simulink model "fish_deboning12"  (R2021a)
settings: Solver=VariableStepAuto  StartTime=0.0  StopTime=10.0  RelTol=1e-3  AbsTol=1e-3
libraries: fl_lib x47, ee_lib x44, nesl_utility x5
settings Model: Creator=Shivu  LastModifiedBy=Shivu
settings SolverCC: AutoScaleAbsTol=off  AlgebraicLoopSolver=TrustRegion
settings DebuggingCC: SymbolicDimsDataTypeCodeGenerationDiagnostic=none  SFMachineParentedDataDiag=warning
settings SFSimCC: CustomCodeUndefinedFunction=UseInterfaceOnly
settings SimscapeCC: SimscapeLogType=all  SimscapeLogSimulationStatistics=on  SimscapeLogDataHistory=10000

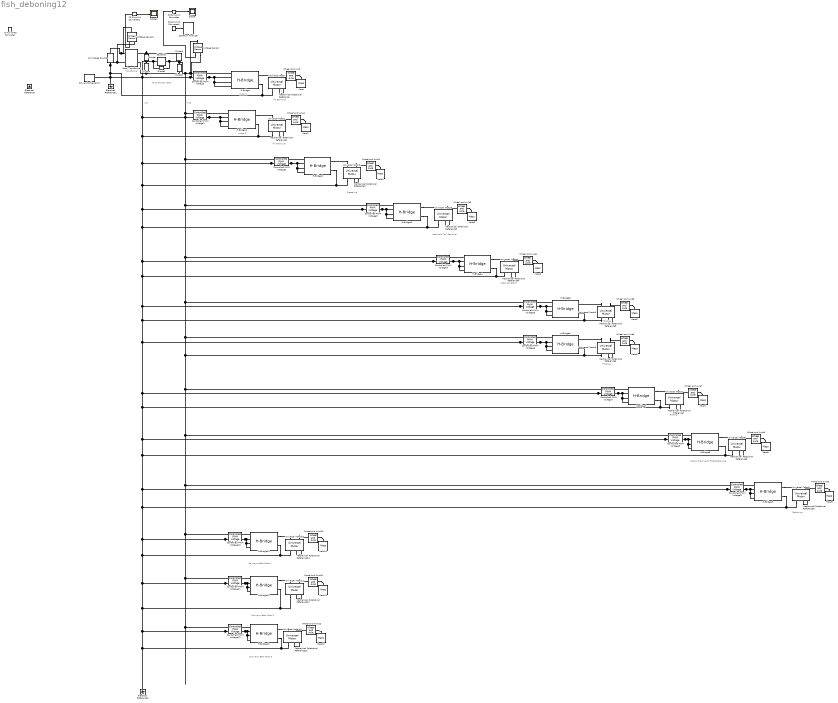
== system fish_deboning12 ==
  note: Conveyor Belt Motor 3
  note: Conveyor Belt Motor 2
  note: Conveyor Belt Motor 1
  note: Deboning
  note: Option flipping for Fillet/Deboning
  note: Gutting
  note: Filleting
  note: Filleting
  note: Head Collection
  note: Head and Tail Removal
  note: Descaling
  note: Fin Removal
  note: Fin Removal
  note: motor 2
  note: motor 1
  note: Transformer
  note: AC to DC Convertor
  note: +VE
  note: -VE
  AC Voltage Source : fl_lib/Electrical/Electrical Sources/AC Voltage Source  amp=230 V  shift=0 deg  frequency=50 Hz  omega=0 rad/s
  Capacitor : fl_lib/Electrical/Electrical Elements/Capacitor  c=4700 uF  r=1e-6 Ohm  g=0 1/Ohm  i_specify=off  i_priority=None  i=0 A  i_nominal_specify=off  i_nominal_unit=A  i_nominal_value=1  v_specify=on  v_priority=High  v=50 V  v_nominal_specify=off  v_nominal_unit=V  v_nominal_value=1  vc_specify=off  vc_priority=Low  vc=0 V  vc_nominal_specify=off  vc_nominal_unit=V  vc_nominal_value=1
  Controlled PWM Voltage{,1..12} (13 alike) : ee_lib/Integrated Circuits/Controlled PWM Voltage  F=1000 Hz  TD=0 s  pulse_width_offset=0 s  pulse_min=0 s  Vmin=0 V  Vmax=230 V  Vm=5 V  pwm_or_av=2  event_type=1  sample_time=1e-6 s  u_min=0  u_max=1
  Diode{,2..4} (4 alike) : ee_lib/Semiconductors & Converters/Diode  ModelType=ee.enum.diode.modelType.pwl  IfMat=[.07, .12, .19, 1.75, 4.24, 7.32, 11.2; .16, .3, .72, 2.14, 4.02, 6.35, 9.12] A  TjVec=[25, 125] degC  VfVec=[.5, .7, .9, 1.3, 1.7, 2.1, 2.5] V  Vf=1.1 V  Ron=0.3 Ohm  Goff=1e-8 S  prmExp=ee.enum.diode.expParam.useTwo  I12=[.0137, .545] A  V12=[.6, .7] V  IS=1e-12 A  ec=1  I1=0.0137 A  V1=0.6 V  RS=0 Ohm  Tmeas=25 degC  N_series=1  N_parallel=1  Rz=0.3 Ohm  BV=inf V  C_param=ee.enum.diode.capParam.fixed  CJ=5 pF  CJ0=5 pF  VJ=1 V  Mgrad=0.5  Vvec=[.1, 10, 100] V  Cvec=[3.5, 1, .4] pF  FC=0.5  Q_param=ee.enum.diode.recoveryParam.off  iRM=-7.15 A  iF=4 A  didt=-750 A/us  trr_factor=3  trr=115 ns  Qrr=150 s*nA  TT=50 ns  tau=100 ns  T_param=ee.enum.diode.temperatureParam.off  IS_T2=1.25e-7 A  I1_T2=0.245 A  V1_T2=0.5 V  Tmeas2=125 degC  EG_param=ee.enum.diode.egapParam.material_si  EG=1.11 eV  XTI_param=ee.enum.diode.xtiParam.pn  XTI=3  dBVdT=0 V/K  enable_faults=ee.enum.faults.faultEnable.no  fault_action=ee.enum.faults.faultAction.none  fault_types=ee.enum.diode.faults.open  tau_fault=1e-3 s  IfMat_faulted=[.07, .12, .19, 1.75, 4.24, 7.32, 11.2; .16, .3, .72, 2.14, 4.02, 6.35, 9.12] A  VfVec_faulted=[.5, .7, .9, 1.3, 1.7, 2.1, 2.5] V  Ropen_faulted=1000 Ohm  Gshort_faulted=1000 1/Ohm  Vf_faulted=0.6 V  Ron_faulted=0.3 Ohm  Goff_faulted=1e-8 S  I12_faulted=[.0137, .545] A  V12_faulted=[.6, .7] V  IS_faulted=1e-12 A  ec_faulted=1  I1_faulted=0.0137 A  V1_faulted=0.6 V  RS_faulted=0 Ohm  Rz_faulted=0.3 Ohm  BV_faulted=inf V  Cscale_faulted=100  enable_temporal_fault=ee.enum.faults.faultEnable.no  t_fault=inf s  enable_behavioral_fault=ee.enum.faults.faultEnable.no  max_permissible_voltage=inf V  n_fail_on_voltage=1  max_permissible_current=inf A  t_fail_on_current=1 s  max_permissible_dVdt=inf V/s  Tdevice=25 degC  i_specify=off  i_priority=None  i=0 A  i_nominal_specify=off  i_nominal_unit=A  i_nominal_value=1  v_specify=off  v_priority=None  v=0 V  v_nominal_specify=off  v_nominal_unit=V  v_nominal_value=1  i_diode_specify=off  i_diode_priority=None  i_diode=0 A  i_diode_nominal_specify=off  i_diode_nominal_unit=A  i_diode_nominal_value=1  v_diode_specify=off  v_diode_priority=None  v_diode=0 V  v_diode_nominal_specify=off  v_diode_nominal_unit=V  v_diode_nominal_value=1  i_capacitor_specify=off  i_capacitor_priority=None  i_capacitor=0 A  i_capacitor_nominal_specify=off  i_capacitor_nominal_unit=A  i_capacitor_nominal_value=1  v_capacitor_specify=off  v_capacitor_priority=None  v_capacitor=0 V  v_capacitor_nominal_specify=off  v_capacitor_nominal_unit=V  v_capacitor_nominal_value=1  power_dissipated_specify=off  power_dissipated_priority=None  power_dissipated=0 W  power_dissipated_nominal_specify=off  power_dissipated_nominal_unit=W  power_dissipated_nominal_value=1  max_permissible_temperature=inf K  t_fail_on_temperature=1 s  thermal_network_parameterization=ee.enum.thermalNetworkTopology.cauer  Rth=[0, 10] K/W  Rth_Foster=[4, 6] K/W  thermal_mass_parameterization=ee.enum.thermalNetwork.timeconstant  thermal_mass=[0, 1] J/K  thermal_mass_Foster=[1.5, 3] J/K  thermal_time_constant=[0, 10] s  thermal_time_constant_Foster=[6, 18] s  thermal_mass_initial_temperatures=[25, 25] degC
  Diode1 : ee_lib/Semiconductors & Converters/Diode  ModelType=ee.enum.diode.modelType.pwl  IfMat=[.07, .12, .19, 1.75, 4.24, 7.32, 11.2; .16, .3, .72, 2.14, 4.02, 6.35, 9.12] A  TjVec=[25, 125] degC  VfVec=[.5, .7, .9, 1.3, 1.7, 2.1, 2.5] V  Vf=0.6 V  Ron=0.3 Ohm  Goff=1e-8 S  prmExp=ee.enum.diode.expParam.useTwo  I12=[.0137, .545] A  V12=[.6, .7] V  IS=1e-12 A  ec=1  I1=0.0137 A  V1=0.6 V  RS=0 Ohm  Tmeas=25 degC  N_series=1  N_parallel=1  Rz=0.3 Ohm  BV=inf V  C_param=ee.enum.diode.capParam.fixed  CJ=5 pF  CJ0=5 pF  VJ=1 V  Mgrad=0.5  Vvec=[.1, 10, 100] V  Cvec=[3.5, 1, .4] pF  FC=0.5  Q_param=ee.enum.diode.recoveryParam.off  iRM=-7.15 A  iF=4 A  didt=-750 A/us  trr_factor=3  trr=115 ns  Qrr=150 s*nA  TT=50 ns  tau=100 ns  T_param=ee.enum.diode.temperatureParam.off  IS_T2=1.25e-7 A  I1_T2=0.245 A  V1_T2=0.5 V  Tmeas2=125 degC  EG_param=ee.enum.diode.egapParam.material_si  EG=1.11 eV  XTI_param=ee.enum.diode.xtiParam.pn  XTI=3  dBVdT=0 V/K  enable_faults=ee.enum.faults.faultEnable.no  fault_action=ee.enum.faults.faultAction.none  fault_types=ee.enum.diode.faults.open  tau_fault=1e-3 s  IfMat_faulted=[.07, .12, .19, 1.75, 4.24, 7.32, 11.2; .16, .3, .72, 2.14, 4.02, 6.35, 9.12] A  VfVec_faulted=[.5, .7, .9, 1.3, 1.7, 2.1, 2.5] V  Ropen_faulted=1000 Ohm  Gshort_faulted=1000 1/Ohm  Vf_faulted=0.6 V  Ron_faulted=0.3 Ohm  Goff_faulted=1e-8 S  I12_faulted=[.0137, .545] A  V12_faulted=[.6, .7] V  IS_faulted=1e-12 A  ec_faulted=1  I1_faulted=0.0137 A  V1_faulted=0.6 V  RS_faulted=0 Ohm  Rz_faulted=0.3 Ohm  BV_faulted=inf V  Cscale_faulted=100  enable_temporal_fault=ee.enum.faults.faultEnable.no  t_fault=inf s  enable_behavioral_fault=ee.enum.faults.faultEnable.no  max_permissible_voltage=inf V  n_fail_on_voltage=1  max_permissible_current=inf A  t_fail_on_current=1 s  max_permissible_dVdt=inf V/s  Tdevice=25 degC  i_specify=off  i_priority=None  i=0 A  i_nominal_specify=off  i_nominal_unit=A  i_nominal_value=1  v_specify=off  v_priority=None  v=0 V  v_nominal_specify=off  v_nominal_unit=V  v_nominal_value=1  i_diode_specify=off  i_diode_priority=None  i_diode=0 A  i_diode_nominal_specify=off  i_diode_nominal_unit=A  i_diode_nominal_value=1  v_diode_specify=off  v_diode_priority=None  v_diode=0 V  v_diode_nominal_specify=off  v_diode_nominal_unit=V  v_diode_nominal_value=1  i_capacitor_specify=off  i_capacitor_priority=None  i_capacitor=0 A  i_capacitor_nominal_specify=off  i_capacitor_nominal_unit=A  i_capacitor_nominal_value=1  v_capacitor_specify=off  v_capacitor_priority=None  v_capacitor=0 V  v_capacitor_nominal_specify=off  v_capacitor_nominal_unit=V  v_capacitor_nominal_value=1  power_dissipated_specify=off  power_dissipated_priority=None  power_dissipated=0 W  power_dissipated_nominal_specify=off  power_dissipated_nominal_unit=W  power_dissipated_nominal_value=1  max_permissible_temperature=inf K  t_fail_on_temperature=1 s  thermal_network_parameterization=ee.enum.thermalNetworkTopology.cauer  Rth=[0, 10] K/W  Rth_Foster=[4, 6] K/W  thermal_mass_parameterization=ee.enum.thermalNetwork.timeconstant  thermal_mass=[0, 1] J/K  thermal_mass_Foster=[1.5, 3] J/K  thermal_time_constant=[0, 10] s  thermal_time_constant_Foster=[6, 18] s  thermal_mass_initial_temperatures=[25, 25] degC
  Electrical Reference : fl_lib/Electrical/Electrical Elements/Electrical Reference
  Electrical Reference1 : fl_lib/Electrical/Electrical Elements/Electrical Reference
  Electrical Reference2 : fl_lib/Electrical/Electrical Elements/Electrical Reference
  H-Bridge{,1..3,5..7,10..12} (10 alike) : ee_lib/Semiconductors & Converters/Converters/H-Bridge  supply_ports=ee.enum.supply_ports.hidesupply  Venable=2.5 V  Vmax=5 V  Vreverse=2.5 V  Vbrake=2.5 V  Vm=13.5 V  pwm_or_av=ee.enum.pwm_or_av.averaged  regenerative_braking_mode=ee.enum.converters.regenerative_braking_mode.depends_on_rev  discontinuous=ee.enum.current_profile.continuous  freewheeling_mode=ee.enum.converters.freewheeling_mode.one_switch_one_diode  Ron=0.1 Ohm  Don=0.05 Ohm  Goff=1e-6 S  Rload=10 Ohm  Lload=1e-5 H  F=10 kHz  thermal_mass=100 J/K  initial_temperature=298.15 K  Ron2=0.1 Ohm  Don2=0.05 Ohm  Tmeas=298.15 K  Tmeas2=398.15 K
  H-Bridge4 : ee_lib/Semiconductors & Converters/Converters/H-Bridge  supply_ports=ee.enum.supply_ports.hidesupply  Venable=2.5 V  Vmax=5 V  Vreverse=2.5 V  Vbrake=2.5 V  Vm=5 V  pwm_or_av=ee.enum.pwm_or_av.averaged  regenerative_braking_mode=ee.enum.converters.regenerative_braking_mode.depends_on_rev  discontinuous=ee.enum.current_profile.continuous  freewheeling_mode=ee.enum.converters.freewheeling_mode.one_switch_one_diode  Ron=0.1 Ohm  Don=0.05 Ohm  Goff=1e-6 S  Rload=10 Ohm  Lload=1e-5 H  F=10 kHz  thermal_mass=100 J/K  initial_temperature=298.15 K  Ron2=0.1 Ohm  Don2=0.05 Ohm  Tmeas=298.15 K  Tmeas2=398.15 K
  H-Bridge8 : ee_lib/Semiconductors & Converters/Converters/H-Bridge  supply_ports=ee.enum.supply_ports.hidesupply  Venable=2.5 V  Vmax=5 V  Vreverse=2.5 V  Vbrake=2.5 V  Vm=5 V  pwm_or_av=ee.enum.pwm_or_av.averaged  regenerative_braking_mode=ee.enum.converters.regenerative_braking_mode.depends_on_rev  discontinuous=ee.enum.current_profile.continuous  freewheeling_mode=ee.enum.converters.freewheeling_mode.one_switch_one_diode  Ron=0.1 Ohm  Don=0.05 Ohm  Goff=1e-6 S  Rload=10 Ohm  Lload=1e-5 H  F=10 kHz  thermal_mass=100 J/K  initial_temperature=298.15 K  Ron2=0.1 Ohm  Don2=0.05 Ohm  Tmeas=298.15 K  Tmeas2=398.15 K
  H-Bridge9 : ee_lib/Semiconductors & Converters/Converters/H-Bridge  supply_ports=ee.enum.supply_ports.hidesupply  Venable=2.5 V  Vmax=5 V  Vreverse=2.5 V  Vbrake=2.5 V  Vm=230 V  pwm_or_av=ee.enum.pwm_or_av.averaged  regenerative_braking_mode=ee.enum.converters.regenerative_braking_mode.depends_on_rev  discontinuous=ee.enum.current_profile.continuous  freewheeling_mode=ee.enum.converters.freewheeling_mode.one_switch_one_diode  Ron=0.1 Ohm  Don=0.05 Ohm  Goff=1e-6 S  Rload=10 Ohm  Lload=1e-5 H  F=10 kHz  thermal_mass=100 J/K  initial_temperature=298.15 K  Ron2=0.1 Ohm  Don2=0.05 Ohm  Tmeas=298.15 K  Tmeas2=398.15 K
  Ideal Transformer : fl_lib/Electrical/Electrical Elements/Ideal Transformer  n=1  i1_specify=off  i1_priority=None  i1=0 A  i1_nominal_specify=off  i1_nominal_unit=A  i1_nominal_value=1  v1_specify=on  v1_priority=High  v1=220 V  v1_nominal_specify=off  v1_nominal_unit=V  v1_nominal_value=1  i2_specify=on  i2_priority=High  i2=1 A  i2_nominal_specify=off  i2_nominal_unit=A  i2_nominal_value=1  v2_specify=on  v2_priority=High  v2=12 V  v2_nominal_specify=off  v2_nominal_unit=V  v2_nominal_value=1
      settings: SourceProductBaseCode=SS
  Mass{,1..12} (13 alike) : fl_lib/Mechanical/Translational Elements/Mass  mass=1 kg  num_ports=foundation.enum.numPorts2.one  v_specify=off  v_priority=High  v=0 m/s  v_nominal_specify=off  v_nominal_unit=m/s  v_nominal_value=1  f_specify=off  f_priority=None  f=0 N  f_nominal_specify=off  f_nominal_unit=N  f_nominal_value=1
  Mechanical Rotational Reference{,1..12} (13 alike) : fl_lib/Mechanical/Rotational Elements/Mechanical Rotational Reference
  PS-Simulink Converter : nesl_utility/PS-Simulink Converter  PhysicalDomain=network_engine_domain  SubClassName=ps_output  LeftPortType=input  RightPortType=output  PseudoPeriodic=off  Frequencies=[]  Unit=inherit  AffineConversion=off
      settings: SourceProductBaseCode=PW,SS
  PS-Simulink Converter1 : nesl_utility/PS-Simulink Converter  PhysicalDomain=network_engine_domain  SubClassName=ps_output  LeftPortType=input  RightPortType=output  PseudoPeriodic=off  Frequencies=[]  Unit=inherit  AffineConversion=off
      settings: SourceProductBaseCode=PW,SS
  PS-Simulink Converter2 : nesl_utility/PS-Simulink Converter  PhysicalDomain=network_engine_domain  SubClassName=ps_output  LeftPortType=input  RightPortType=output  PseudoPeriodic=off  Frequencies=[]  Unit=inherit  AffineConversion=off
      settings: SourceProductBaseCode=PW,SS
  Scope : Scope
  Scope1 : Scope
  Simulink-PS Converter : nesl_utility/Simulink-PS Converter  PhysicalDomain=network_engine_domain  SubClassName=ps_input  LeftPortType=input  RightPortType=output  PseudoPeriodic=off  Frequencies=[]  NoiseDistribution=none  NoiseParameters=[]  Unit=1  AffineConversion=off  FilteringAndDerivatives=provide  SimscapeFilterOrder=1  InputFilterTimeConstant=0.001  UdotUserProvided=0
      settings: SourceProductBaseCode=PW,SS
  Solver Configuration : nesl_utility/Solver Configuration  PhysicalDomain=network_engine_domain  SubClassName=solver  LeftPortType=input  RightPortType=generic  Tones=[]  Harmonics=[]  SimulateNoise=off  Profile=off  UseLocalSampling=off  EnableSwitchedLinearOptims=on  FrequencyDomain=off  UseCCode=off  RelTol=0.001  AbsTol=1e-06  MinStep=1e-09  ToWorkspace=off  RevertToSquareIcSolve=off  NumHomotopyIterations=100  PhasorMode=off  PhasorModeNumHarmonics=1  DoDC=off  ResidualTolerance=1e-09  UseLocalSolver=off  LocalSolverChoice=NE_BACKWARD_EULER_ADVANCER  LocalSolverSampleTime=0.001  DoFixedCost=off  MaxNonlinIter=3  MaxModeIter=2  ComputeImpulses=off  ImpulseIterations=2  LinearAlgebra=auto  EquationFormulation=NE_TIME_EF  DelaysMemoryBudget=1024  AutomaticFiltering=on  FilteringTimeConstant=0.001  PartitionStorageMethod=AS_NEEDED  PartitionMemoryBudget=1024  PartitionMethod=ROBUST
      settings: SourceProductBaseCode=PW,SS
  Spectrum Analyzer : SpectrumAnalyzer
  Universal Motor{,1..3,5..7,10..12} (10 alike) : ee_lib/Electromechanical/Brushed Motors/Universal Motor  parameterization=2  Ra=132.8 Ohm  Laf=0.1722 s*V/rad/A  w_rated=6500 rpm  P_rated=100 W  V_dc=12 V  T_max=5 N*m  P_in=160 W  V_ac=240 V  I_ac=0.8 A  w_ac=50 Hz  Ltot=0.525 H  J=2e-4 kg*m^2  lam=1e-6 N*m/(rad/s)  speed0=0 rpm  resistance_ratio=1  alpha=[.00393, .00393] 1/K  Tmeas=25 degC  thermal_masses=[100, 100] J/K  initial_temperatures=[25, 25] degC
      settings: SourceProductBaseCode=PS  InternalSimscapePortConfiguration="{\"Bottom\":[],\"Left\":[{\"id\":\"p\",\"label\":\"+\",\"type\":\"foundation.electrical.electrical\"},{\"id\":\"R\",\"label\":\"R\",\"type\":\"foundation.mechanical.rotational.rotational\"}],\"Right\":[{\"id\":\"n\",\"label\":\"-\",\"type\":\"foundation.electrical.electrical\"},{\"id\":\"C\",\"label\":\"C\",\"type\":\"foundation.mechanical.rotational.rotational\"}],\"Top\":[]}"
  Universal Motor4 : ee_lib/Electromechanical/Brushed Motors/Universal Motor  parameterization=2  Ra=132.8 Ohm  Laf=0.1722 s*V/rad/A  w_rated=300 rpm  P_rated=100 W  V_dc=36 V  T_max=5 N*m  P_in=160 W  V_ac=240 V  I_ac=0.8 A  w_ac=50 Hz  Ltot=0.525 H  J=2e-4 kg*m^2  lam=1e-6 N*m/(rad/s)  speed0=0 rpm  resistance_ratio=1  alpha=[.00393, .00393] 1/K  Tmeas=25 degC  thermal_masses=[100, 100] J/K  initial_temperatures=[25, 25] degC
      settings: SourceProductBaseCode=PS  InternalSimscapePortConfiguration="{\"Bottom\":[],\"Left\":[{\"id\":\"p\",\"label\":\"+\",\"type\":\"foundation.electrical.electrical\"},{\"id\":\"R\",\"label\":\"R\",\"type\":\"foundation.mechanical.rotational.rotational\"}],\"Right\":[{\"id\":\"n\",\"label\":\"-\",\"type\":\"foundation.electrical.electrical\"},{\"id\":\"C\",\"label\":\"C\",\"type\":\"foundation.mechanical.rotational.rotational\"}],\"Top\":[]}"
  Universal Motor8 : ee_lib/Electromechanical/Brushed Motors/Universal Motor  parameterization=2  Ra=132.8 Ohm  Laf=0.1722 s*V/rad/A  w_rated=300 rpm  P_rated=100 W  V_dc=36 V  T_max=5 N*m  P_in=160 W  V_ac=240 V  I_ac=0.8 A  w_ac=50 Hz  Ltot=0.525 H  J=2e-4 kg*m^2  lam=1e-6 N*m/(rad/s)  speed0=0 rpm  resistance_ratio=1  alpha=[.00393, .00393] 1/K  Tmeas=25 degC  thermal_masses=[100, 100] J/K  initial_temperatures=[25, 25] degC
      settings: SourceProductBaseCode=PS  InternalSimscapePortConfiguration="{\"Bottom\":[],\"Left\":[{\"id\":\"p\",\"label\":\"+\",\"type\":\"foundation.electrical.electrical\"},{\"id\":\"R\",\"label\":\"R\",\"type\":\"foundation.mechanical.rotational.rotational\"}],\"Right\":[{\"id\":\"n\",\"label\":\"-\",\"type\":\"foundation.electrical.electrical\"},{\"id\":\"C\",\"label\":\"C\",\"type\":\"foundation.mechanical.rotational.rotational\"}],\"Top\":[]}"
  Universal Motor9 : ee_lib/Electromechanical/Brushed Motors/Universal Motor  parameterization=2  Ra=132.8 Ohm  Laf=0.1722 s*V/rad/A  w_rated=1500 rpm  P_rated=100 W  V_dc=220 V  T_max=5 N*m  P_in=160 W  V_ac=240 V  I_ac=0.8 A  w_ac=50 Hz  Ltot=0.525 H  J=2e-4 kg*m^2  lam=1e-6 N*m/(rad/s)  speed0=0 rpm  resistance_ratio=1  alpha=[.00393, .00393] 1/K  Tmeas=25 degC  thermal_masses=[100, 100] J/K  initial_temperatures=[25, 25] degC
      settings: SourceProductBaseCode=PS  InternalSimscapePortConfiguration="{\"Bottom\":[],\"Left\":[{\"id\":\"p\",\"label\":\"+\",\"type\":\"foundation.electrical.electrical\"},{\"id\":\"R\",\"label\":\"R\",\"type\":\"foundation.mechanical.rotational.rotational\"}],\"Right\":[{\"id\":\"n\",\"label\":\"-\",\"type\":\"foundation.electrical.electrical\"},{\"id\":\"C\",\"label\":\"C\",\"type\":\"foundation.mechanical.rotational.rotational\"}],\"Top\":[]}"
  Voltage Sensor : fl_lib/Electrical/Electrical Sensors/Voltage Sensor
  Voltage Sensor1 : fl_lib/Electrical/Electrical Sensors/Voltage Sensor
  Wheel and Axle{,1..12} (13 alike) : fl_lib/Mechanical/Mechanisms/Wheel and Axle  R=0.05 m  or=1  t_specify=off  t_priority=None  t=0 N*m  t_nominal_specify=off  t_nominal_unit=N*m  t_nominal_value=1  f_specify=off  f_priority=None  f=0 N  f_nominal_specify=off  f_nominal_unit=N  f_nominal_value=1
  wires:
  PS-Simulink Converter/1 -> Scope/1
  PS-Simulink Converter1/1 -> Spectrum Analyzer/1
  PS-Simulink Converter2/1 -> Scope1/1
  connections:
  AC Voltage Source/LConn1 -- Voltage Sensor1/LConn1 -- Ideal Transformer/LConn1
  Controlled PWM Voltage/RConn2 -- H-Bridge/LConn2 -- H-Bridge/LConn4 -- H-Bridge/LConn3 -- Electrical Reference1/LConn1 -- Solver Configuration/RConn1 -- Universal Motor/RConn1 -- H-Bridge/RConn2 -- AC Voltage Source/RConn1 -- Voltage Sensor1/RConn2 -- Ideal Transformer/LConn2
  H-Bridge12/LConn2 -- H-Bridge12/LConn4 -- H-Bridge12/LConn3 -- H-Bridge12/RConn2 -- Universal Motor12/RConn1 -- Electrical Reference2/LConn1 -- H-Bridge11/RConn2 -- Universal Motor11/RConn1 -- Controlled PWM Voltage11/RConn2 -- H-Bridge11/LConn4 -- H-Bridge11/LConn3 -- H-Bridge11/LConn2 -- Controlled PWM Voltage11/LConn2 -- H-Bridge10/RConn2 -- Universal Motor10/RConn1 -- H-Bridge10/LConn2 -- H-Bridge10/LConn4 -- H-Bridge10/LConn3 -- Controlled PWM Voltage10/RConn2 -- Controlled PWM Voltage10/LConn2 -- H-Bridge9/RConn2 -- Universal Motor9/RConn1 -- H-Bridge9/LConn4 -- H-Bridge9/LConn3 -- H-Bridge9/LConn2 -- Controlled PWM Voltage9/RConn2 -- Controlled PWM Voltage9/LConn2 -- H-Bridge8/RConn2 -- Universal Motor8/RConn1 -- H-Bridge8/LConn4 -- H-Bridge8/LConn3 -- H-Bridge8/LConn2 -- Controlled PWM Voltage8/RConn2 -- Controlled PWM Voltage8/LConn2 -- H-Bridge7/RConn2 -- Universal Motor7/RConn1 -- H-Bridge7/LConn4 -- H-Bridge7/LConn3 -- H-Bridge7/LConn2 -- Controlled PWM Voltage7/RConn2 -- Controlled PWM Voltage7/LConn2 -- H-Bridge6/LConn4 -- H-Bridge6/LConn3 -- H-Bridge6/LConn2 -- Controlled PWM Voltage6/RConn2 -- Controlled PWM Voltage6/LConn2 -- H-Bridge5/RConn2 -- Universal Motor5/RConn1 -- H-Bridge5/LConn4 -- H-Bridge5/LConn3 -- H-Bridge5/LConn2 -- Controlled PWM Voltage5/RConn2 -- Controlled PWM Voltage5/LConn2 -- H-Bridge4/RConn2 -- Universal Motor4/RConn1 -- H-Bridge4/LConn4 -- H-Bridge4/LConn3 -- H-Bridge4/LConn2 -- Controlled PWM Voltage4/RConn2 -- Controlled PWM Voltage4/LConn2 -- H-Bridge3/LConn4 -- H-Bridge3/LConn3 -- H-Bridge3/LConn2 -- Controlled PWM Voltage3/RConn2 -- Controlled PWM Voltage3/LConn2 -- H-Bridge2/RConn2 -- Universal Motor2/RConn1 -- H-Bridge2/LConn4 -- H-Bridge2/LConn3 -- H-Bridge2/LConn2 -- Controlled PWM Voltage2/RConn2 -- Controlled PWM Voltage2/LConn2 -- Voltage Sensor/RConn2 -- Controlled PWM Voltage/LConn2 -- Diode4/LConn1 -- Diode1/LConn1 -- Capacitor/RConn1 -- Diode/LConn1 -- Controlled PWM Voltage1/LConn2 -- H-Bridge1/RConn2 -- Universal Motor1/RConn1 -- H-Bridge3/RConn2 -- Universal Motor3/RConn1 -- Controlled PWM Voltage12/LConn2 -- Controlled PWM Voltage12/RConn2
  Diode/RConn1 -- Diode3/LConn1 -- Ideal Transformer/RConn1
  Diode4/RConn1 -- Diode2/LConn1 -- Ideal Transformer/RConn2
  H-Bridge/LConn1 -- Controlled PWM Voltage/RConn1
  Universal Motor/LConn1 -- H-Bridge/RConn1
  Universal Motor/RConn2 -- Mechanical Rotational Reference/LConn1
  Universal Motor/LConn2 -- Wheel and Axle/LConn1
  Wheel and Axle/RConn1 -- Mass/LConn1
  Controlled PWM Voltage1/RConn2 -- H-Bridge1/LConn4 -- H-Bridge1/LConn3 -- H-Bridge1/LConn2 -- Controlled PWM Voltage1/LConn1 -- Voltage Sensor/LConn1 -- Controlled PWM Voltage/LConn1 -- Diode2/RConn1 -- Diode1/RConn1 -- Capacitor/LConn1 -- Diode3/RConn1 -- Controlled PWM Voltage2/LConn1 -- Controlled PWM Voltage4/LConn1 -- H-Bridge6/RConn2 -- Universal Motor6/RConn1 -- Controlled PWM Voltage7/LConn1 -- Controlled PWM Voltage9/LConn1 -- Controlled PWM Voltage12/LConn1 -- Controlled PWM Voltage11/LConn1 -- Controlled PWM Voltage10/LConn1 -- Controlled PWM Voltage8/LConn1 -- Controlled PWM Voltage6/LConn1 -- Controlled PWM Voltage5/LConn1 -- Controlled PWM Voltage3/LConn1
  Voltage Sensor/RConn1 -- PS-Simulink Converter/LConn1
  Controlled PWM Voltage1/RConn1 -- H-Bridge1/LConn1
  H-Bridge1/RConn1 -- Universal Motor1/LConn1
  Mechanical Rotational Reference1/LConn1 -- Universal Motor1/RConn2
  Wheel and Axle1/RConn1 -- Mass1/LConn1
  Universal Motor1/LConn2 -- Wheel and Axle1/LConn1
  H-Bridge2/LConn1 -- Controlled PWM Voltage2/RConn1
  H-Bridge2/RConn1 -- Universal Motor2/LConn1
  Universal Motor2/LConn2 -- Wheel and Axle2/LConn1
  Mechanical Rotational Reference2/LConn1 -- Universal Motor2/RConn2
  Wheel and Axle2/RConn1 -- Mass2/LConn1
  H-Bridge3/LConn1 -- Controlled PWM Voltage3/RConn1
  Wheel and Axle3/RConn1 -- Mass3/LConn1
  Universal Motor3/LConn2 -- Wheel and Axle3/LConn1
  Mechanical Rotational Reference3/LConn1 -- Universal Motor3/RConn2
  H-Bridge3/RConn1 -- Universal Motor3/LConn1
  H-Bridge4/LConn1 -- Controlled PWM Voltage4/RConn1
  H-Bridge4/RConn1 -- Universal Motor4/LConn1
  Universal Motor4/LConn2 -- Wheel and Axle4/LConn1
  Mechanical Rotational Reference4/LConn1 -- Universal Motor4/RConn2
  Wheel and Axle4/RConn1 -- Mass4/LConn1
  Wheel and Axle5/RConn1 -- Mass5/LConn1
  Mechanical Rotational Reference5/LConn1 -- Universal Motor5/RConn2
  Universal Motor5/LConn2 -- Wheel and Axle5/LConn1
  H-Bridge5/LConn1 -- Controlled PWM Voltage5/RConn1
  Universal Motor5/LConn1 -- H-Bridge5/RConn1
  H-Bridge6/LConn1 -- Controlled PWM Voltage6/RConn1
  Universal Motor6/LConn2 -- Wheel and Axle6/LConn1
  Wheel and Axle6/RConn1 -- Mass6/LConn1
  Universal Motor6/LConn1 -- H-Bridge6/RConn1
  Mechanical Rotational Reference6/LConn1 -- Universal Motor6/RConn2
  Voltage Sensor1/RConn1 -- PS-Simulink Converter2/LConn1
  H-Bridge7/LConn1 -- Controlled PWM Voltage7/RConn1
  Wheel and Axle7/RConn1 -- Mass7/LConn1
  Universal Motor7/LConn2 -- Wheel and Axle7/LConn1
  Mechanical Rotational Reference7/LConn1 -- Universal Motor7/RConn2
  H-Bridge7/RConn1 -- Universal Motor7/LConn1
  H-Bridge8/LConn1 -- Controlled PWM Voltage8/RConn1
  Mechanical Rotational Reference8/LConn1 -- Universal Motor8/RConn2
  Universal Motor8/LConn2 -- Wheel and Axle8/LConn1
  Wheel and Axle8/RConn1 -- Mass8/LConn1
  H-Bridge8/RConn1 -- Universal Motor8/LConn1
  H-Bridge9/LConn1 -- Controlled PWM Voltage9/RConn1
  Universal Motor9/LConn2 -- Wheel and Axle9/LConn1
  Mechanical Rotational Reference9/LConn1 -- Universal Motor9/RConn2
  Wheel and Axle9/RConn1 -- Mass9/LConn1
  H-Bridge9/RConn1 -- Universal Motor9/LConn1
  Mechanical Rotational Reference10/LConn1 -- Universal Motor10/RConn2
  Universal Motor10/LConn2 -- Wheel and Axle10/LConn1
  Wheel and Axle10/RConn1 -- Mass10/LConn1
  H-Bridge10/LConn1 -- Controlled PWM Voltage10/RConn1
  H-Bridge10/RConn1 -- Universal Motor10/LConn1
  Mechanical Rotational Reference11/LConn1 -- Universal Motor11/RConn2
  Universal Motor11/LConn2 -- Wheel and Axle11/LConn1
  Wheel and Axle11/RConn1 -- Mass11/LConn1
  H-Bridge11/RConn1 -- Universal Motor11/LConn1
  H-Bridge11/LConn1 -- Controlled PWM Voltage11/RConn1
  H-Bridge12/LConn1 -- Controlled PWM Voltage12/RConn1
  Universal Motor12/LConn2 -- Wheel and Axle12/LConn1
  Mechanical Rotational Reference12/LConn1 -- Universal Motor12/RConn2
  Wheel and Axle12/RConn1 -- Mass12/LConn1
  Universal Motor12/LConn1 -- H-Bridge12/RConn1
